simulink model "ExampleMarketMaker"  (R2015a)
settings: Solver=FixedStepDiscrete  SolverMode=SingleTasking  StartTime=0.0  StopTime=49500  RelTol=1e-3
PreLoadFcn:
  | load('MSFTData.mat')
libraries: dspsrcs4 x2
settings Model: Creator=kassama  LastModifiedBy=skozola
settings DataIOCC: SignalLoggingSaveFormat=ModelDataLogs  SaveOutput=off  SignalLogging=off  SaveTime=off
settings OptimizationCC: ExpressionDepthLimit=2147483647  InitFltsAndDblsToZero=on
settings DebuggingCC: AlgebraicLoopMsg=error  UnderspecifiedInitializationDetection=Classic  MergeDetectMultiDrivingBlocksExec=none  SolverPrmCheckMsg=warning  SingleTaskRateTransMsg=error  FcnCallInpInsideContextMsg=UseLocalSettings  StateNameClashWarn=warning
settings SFSimCC: SimParseCustomCode=off
settings GRTTargetCC: CombineOutputUpdateFcns=off  GRTInterface=on

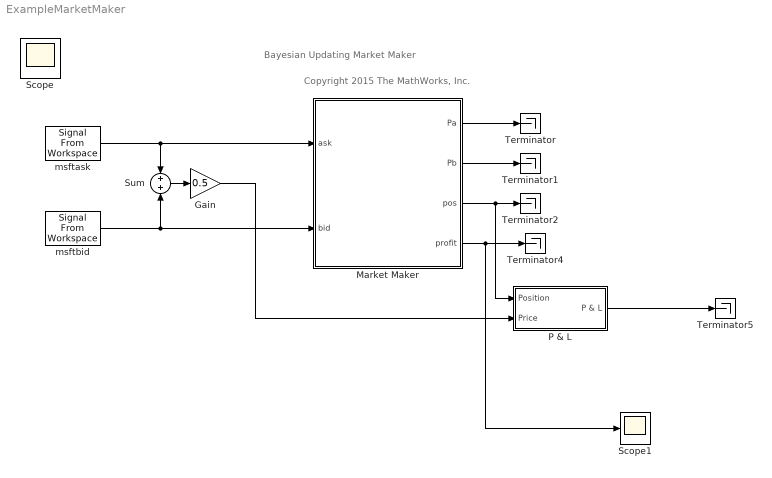
== system ExampleMarketMaker ==
  note: Bayesian Updating Market Maker
  note: Copyright 2015 The MathWorks, Inc.
  Gain : Gain  Gain=0.5
  Market Maker : Stateflow chart  TreatAsAtomicUnit=on
  P & L : Subsystem
  Scope1 : Scope
      settings: YMin=-200  YMax=175  MaxDataPoints=50000
  Sum : Sum
  Terminator{,1..2,4..5} (5 alike) : Terminator
  msftask : dspsrcs4/Signal From Workspace  X=msftask  Ts=1  nsamps=1  OutputAfterFinalValue=Setting to zero  ignoreOrWarnInputAndFrameLengths=off
  msftbid : dspsrcs4/Signal From Workspace  X=msftbid  Ts=1  nsamps=1  OutputAfterFinalValue=Setting to zero  ignoreOrWarnInputAndFrameLengths=off
  Scope : Scope  NumInputPorts=3
      settings: ShowLegends=on  TimeRange=49500  YMin=27.8~-10~-1  YMax=28.8~10~1  MaxDataPoints=7500
  wires:
  msftask/1 -> Market Maker/1(ask), Sum/1
  msftbid/1 -> Market Maker/2(bid), Sum/2
  Market Maker/1(Pa) -> Terminator/1
  Market Maker/2(Pb) -> Terminator1/1
  Market Maker/3(pos) -> Terminator2/1, P & L/1(Position)
  Sum/1 -> Gain/1
  Gain/1 -> P & L/2(Price)
  Market Maker/4(profit) -> Scope1/1, Terminator4/1
  P & L/1(P & L) -> Terminator5/1

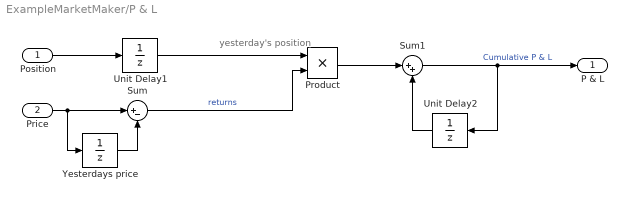
== system ExampleMarketMaker/P & L ==
  note: yesterday's position
  Position : Inport
  Price : Inport  Port=2
  Product : Product  RndMeth=Zero
  Sum : Sum  Inputs=|+-
  Sum1 : Sum  Inputs=|++
  Unit Delay1 : UnitDelay  SampleTime=-1
  Unit Delay2 : UnitDelay  SampleTime=-1
  Yesterdays price : UnitDelay  SampleTime=-1
  P & L : Outport
  wires:
  Sum1/1 -> Unit Delay2/1, P & L/1  "Cumulative P & L"
  Unit Delay2/1 -> Sum1/2
  Yesterdays price/1 -> Sum/2
  Product/1 -> Sum1/1
  Unit Delay1/1 -> Product/1
  Sum/1 -> Product/2  "returns"
  Price/1 -> Yesterdays price/1, Sum/1
  Position/1 -> Unit Delay1/1

== stateflow chart ExampleMarketMaker/Market Maker ==
  state Quote
  (default) -> Quote : {initProb();
      | pos=0; profit = 0;
      | BidAsk();}
  (junction 36) -> Quote : % Inventory control
      | {icontrol();}
  Quote -> (junction 2) [order 2] : % Market buy order
      | [bid >= Pa]
      | {pos = pos - 1;
      | profit = profit + bid;
      | Prob(Pa,1);}
  Quote -> (junction 2) [order 1] : % Market sell order
      | [ask<=Pb]
      | {pos = pos + 1;
      | profit = profit - ask;
      | Prob(Pb,-1);}
  (junction 2) -> (junction 36) : % Recalculate Bid/Ask prices
      | {BidAsk();}
  data: Price function_input double; trade function_input double; ask input; bid input; Pa output double; Pb output double; pos output double; V local double size=[111 1]; P local double size=[111 1]; alpha constant double =0.90; profit output double =0; sigma constant double =0.125
  function BidAsk:
    | function BidAsk()
    | 
    | N=111; 
    | % calculate expected value
    | Eorig = sum(V.*P);
    | % round to nearest cent
    | E = round(Eorig*100)/100;
    | t=0.5+0.5*alpha;
    | % find where E occurs in V
    | %[m,EN]=min(abs(V-E));
    | biderror=zeros(N,1);
    | PB=zeros(N,1);
    | % loop over all values of V from Vmin to E
    | for i=1:N
    |     [PB(i), biderror(i)]=bidCalc(i,V,P,t);
    | end
    | 
    | [minerr,ind]=min(biderror);
    | Pb=min(V(ind),E);
    | 
    | askerror=zeros(N,1);
    | PA=zeros(N,1);
    | % loop over all values of V from E to Vmax
    | for i=1:N
    |     [PA(i), askerror(i)]=askCalc(i,V,P,t);
    | end
    | [minerr,ind]=min(askerror);
    | Pa=max(V(ind), E);
    | 
    | %%% ============================== %%%%
    | function [PB,BidErr]=bidCalc(count,V,P,t)
    | N=length(V);
    | a=0;b=0;
    | for i=1:count
    |     a = a+V(i)*P(i);
    | end
    | 
    | for i=count+1:N
    |     b = b+V(i)*P(i);
    | end
    | PB=2*(t*a + (1-t)*b);
    | BidErr = abs(V(count) - PB);
    | 
    | %%%% ============================ %%%%
    | function [PB,BidErr]=askCalc(count,V,P,t)
    | N=length(V);
    | a=0;b=0;
    | for i=1:count-1
    |     a = a+V(i)*P(i);
    | end
    | 
    | for i=count:N
    |     b = b+V(i)*P(i);
    | end
    | PB=2*((1-t)*a + t*b);
    | BidErr = abs(V(count) - PB);
  function initProb:
    | function initProb()
    | % initial grid of prices
    | 
    | x0 = 28.5850;
    | %x0=27.97;
    | V = (27.9:0.01:29)';
    | 
    | 
    | % normal distn centered around an initial point
    | distn = (1/(sigma*sqrt(2*pi)))*exp(-(V-x0).^2/(2*sigma^2));
    | distn = distn/sum(distn);
    | P = distn;
  function Prob(Price,trade):
    | function Prob(Price,trade)
    | % calculate the probability vector
    | % trade is in [-1 0 1] representing sell, flat, buy orders
    | Pold=P;
    | p=(0.5+0.5*alpha);
    | if trade < 0
    |     % sell order received
    |     for i=1:size(V,1)
    |         if V(i,1) < Price
    |             P(i,1)=Pold(i,1)*p;
    |         else
    |             P(i,1)=Pold(i,1)*(1-p);
    |         end
    |     end
    | else %trade > 0
    |     % buy order received
    |     for i=1:size(V,1)
    |         if V(i) > Price
    |             P(i,1)=Pold(i,1)*p;
    |         else
    |             P(i,1)=Pold(i,1)*(1-p);
    |         end
    |     end
    | end
    | 
    | % normalise
    | P=P/sum(P);
  function icontrol:
    | function icontrol()
    | 
    | % sigmoidal function
    | sig = (10*(1+tanh(-3:0.5:3)));
    | xc= 0:length(sig)-1;
    | 
    | % calculate offset
    | offset = round(sign(pos)*interp1(xc,sig,abs(pos),'linear',max(sig)))/100;
    | %offset=0;
    | if pos>0
    |     Pa=Pa-offset;
    |     Pb=Pb-offset;
    | end
